simulink model "thermal_closed_loop_model"  (R2023a)
settings: Solver=ode23t  StartTime=0.0  StopTime=600  RelTol=1e-3
PostLoadFcn:
  | run('thermal_model_parameters.m')
  | run('thermal_harness_parameters.m')
  | run('thermal_variants_config.m')
values from neighbouring files (symbols this model uses):
  air_cp = 1004    [cathode_subsystem_parameters.m]    (also in thermal_subsystem_parameters.m)
  air_HC_min = 10    [cathode_subsystem_parameters.m]    (also in thermal_subsystem_parameters.m)
  air_HC_nom = 100    [cathode_subsystem_parameters.m]    (also in thermal_subsystem_parameters.m)
  air_rho = 1.2    [cathode_subsystem_parameters.m]    (also in thermal_subsystem_parameters.m)
  air_vel_nom = 1    [cathode_subsystem_parameters.m]    (also in thermal_subsystem_parameters.m)
  coolant_initial_pressure = 0.111325    [cathode_subsystem_parameters.m]    (also in thermal_subsystem_parameters.m)
  coolant_initial_temperature = 293.15    [cathode_subsystem_parameters.m]    (also in thermal_subsystem_parameters.m)
  coolant_tube_D = 0.05    [cathode_subsystem_parameters.m]    (also in thermal_subsystem_parameters.m)
  Hydrowell_VTS =     [Hydrowell_values_VLV.mat]
  radiator_area_air = 0.10260000000000001    (= 0.1026)    [cathode_subsystem_parameters.m]    (also in thermal_subsystem_parameters.m)
  radiator_area_fins = 2.5436250000000005    (= 2.543625)    [cathode_subsystem_parameters.m]    (also in thermal_subsystem_parameters.m)
  radiator_area_primary = 0.44452500000000011    (= 0.444525)    [cathode_subsystem_parameters.m]    (also in thermal_subsystem_parameters.m = 2 * radiator_tube_length * radiator_width * (radiator_fin_ro)
  radiator_n_tubes = 20    [cathode_subsystem_parameters.m]    (also in thermal_subsystem_parameters.m)
  radiator_tube_height = 0.0015    [cathode_subsystem_parameters.m]    (also in thermal_subsystem_parameters.m)
  radiator_tube_length = 0.45    [cathode_subsystem_parameters.m]    (also in thermal_subsystem_parameters.m)
  radiator_width = 0.025    [cathode_subsystem_parameters.m]    (also in thermal_subsystem_parameters.m)
  tcp_time_constant = 2    [cathode_subsystem_parameters.m]    (also in thermal_subsystem_parameters.m)
undefined symbols (not defined in the file or in its folder): sigbuilder_block, stack
libraries: fl_lib x153, nesl_utility x122, SimscapeFluids_lib x16, slpidlib x5, simulink x1
(part 7 of 8)

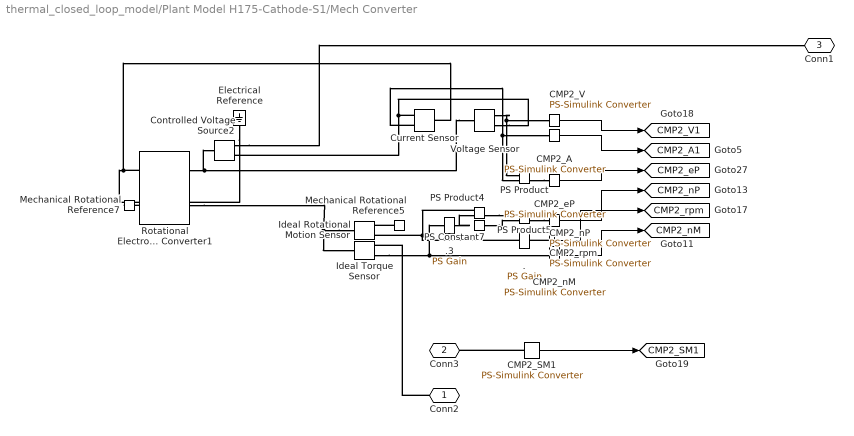
== system thermal_closed_loop_model/Plant Model H175-Cathode-S1/Mech Converter ==
  . : fl_lib/Physical Signals/Functions/PS Gain  gain=1/(0.1047198*1000)
  .3 : fl_lib/Physical Signals/Functions/PS Gain  gain=1/(0.1047198*60)
  CMP2_A : nesl_utility/PS-Simulink Converter  PhysicalDomain=network_engine_domain  SubClassName=ps_output  LeftPortType=input  RightPortType=output  PseudoPeriodic=off  Frequencies=[]  VectorFormat=inherit  Unit=inherit  AffineConversion=off
  CMP2_SM1 : nesl_utility/PS-Simulink Converter  PhysicalDomain=network_engine_domain  SubClassName=ps_output  LeftPortType=input  RightPortType=output  PseudoPeriodic=off  Frequencies=[]  VectorFormat=inherit  Unit=inherit  AffineConversion=off
  CMP2_V : nesl_utility/PS-Simulink Converter  PhysicalDomain=network_engine_domain  SubClassName=ps_output  LeftPortType=input  RightPortType=output  PseudoPeriodic=off  Frequencies=[]  VectorFormat=inherit  Unit=inherit  AffineConversion=off
  CMP2_eP : nesl_utility/PS-Simulink Converter  PhysicalDomain=network_engine_domain  SubClassName=ps_output  LeftPortType=input  RightPortType=output  PseudoPeriodic=off  Frequencies=[]  VectorFormat=inherit  Unit=inherit  AffineConversion=off
  CMP2_nM : nesl_utility/PS-Simulink Converter  PhysicalDomain=network_engine_domain  SubClassName=ps_output  LeftPortType=input  RightPortType=output  PseudoPeriodic=off  Frequencies=[]  VectorFormat=1-D array  Unit=inherit  AffineConversion=off
  CMP2_nP : nesl_utility/PS-Simulink Converter  PhysicalDomain=network_engine_domain  SubClassName=ps_output  LeftPortType=input  RightPortType=output  PseudoPeriodic=off  Frequencies=[]  VectorFormat=inherit  Unit=inherit  AffineConversion=off
  CMP2_rpm : nesl_utility/PS-Simulink Converter  PhysicalDomain=network_engine_domain  SubClassName=ps_output  LeftPortType=input  RightPortType=output  PseudoPeriodic=off  Frequencies=[]  VectorFormat=inherit  Unit=inherit  AffineConversion=off
  Controlled Voltage Source2 : fl_lib/Electrical/Electrical Sources/Controlled Voltage Source
  Current Sensor : fl_lib/Electrical/Electrical Sensors/Current Sensor
  Electrical Reference : fl_lib/Electrical/Electrical Elements/Electrical Reference
  Ideal Rotational Motion Sensor : fl_lib/Mechanical/Mechanical Sensors/Ideal Rotational Motion Sensor  reference=foundation.enum.MeasurementReference.difference  acceleration_port=false  velocity_port=true  position_port=false  wrap_angle=false  offset=0 rad
      settings: InternalSimscapePortConfiguration="{\"Bottom\":[],\"Left\":[{\"id\":\"R\",\"label\":\"R\",\"type\":\"foundation.mechanical.rotational.rotational\"}],\"Right\":[{\"id\":\"C\",\"label\":\"C\",\"type\":\"foundation.mechanical.rotational.rotational\"},{\"id\":\"W\",\"label\":\"W\",\"type\":\"output\"}],\"Top\":[]}"
  Ideal Torque Sensor : fl_lib/Mechanical/Mechanical Sensors/Ideal Torque Sensor
  Mechanical Rotational Reference5 : fl_lib/Mechanical/Rotational Elements/Mechanical Rotational Reference
  Mechanical Rotational Reference7 : fl_lib/Mechanical/Rotational Elements/Mechanical Rotational Reference
  PS Constant7 : fl_lib/Physical Signals/Sources/PS Constant  constant=2*pi
  PS Product : fl_lib/Physical Signals/Functions/PS Product
  PS Product4 : fl_lib/Physical Signals/Functions/PS Product
  PS Product5 : fl_lib/Physical Signals/Functions/PS Product
  Rotational Electromechanical Converter1 : fl_lib/Electrical/Electrical Elements/Rotational Electromechanical Converter  K=0.00409090909090909090909090909091 V/rpm  i_specify=off  i_priority=None  i=0 A  i_nominal_specify=off  i_nominal_unit=A  i_nominal_value=1  v_specify=off  v_priority=None  v=50 V  v_nominal_specify=off  v_nominal_unit=V  v_nominal_value=1  t_specify=off  t_priority=None  t=0 N*m  t_nominal_specify=off  t_nominal_unit=N*m  t_nominal_value=1  w_specify=off  w_priority=None  w=0 rad/s  w_nominal_specify=off  w_nominal_unit=rad/s  w_nominal_value=1
  Voltage Sensor : fl_lib/Electrical/Electrical Sensors/Voltage Sensor
  Conn2 : PMIOPort  Side=Left
  Conn3 : PMIOPort  Port=2  Side=Right
  Conn1 : PMIOPort  Port=3  Side=Right
  tag scope: CMP2_A1=global, CMP2_SM1=global, CMP2_V1=global, CMP2_eP=global, CMP2_nM=global, CMP2_nP=global, CMP2_rpm=global
  wires:
  CMP2_eP/1 -> [CMP2_eP]
  CMP2_V/1 -> [CMP2_V1]
  CMP2_A/1 -> [CMP2_A1]
  CMP2_nM/1 -> [CMP2_nM]
  CMP2_rpm/1 -> [CMP2_rpm]
  CMP2_nP/1 -> [CMP2_nP]
  CMP2_SM1/1 -> [CMP2_SM1]
  connections:
  CMP2_rpm/LConn1 -- ./RConn1
  PS Constant7/RConn1 -- PS Product5/LConn2
  Rotational Electromechanical Converter1/RConn2 -- Mechanical Rotational Reference7/LConn1
  Voltage Sensor/LConn1 -- Controlled Voltage Source2/LConn1 -- Rotational Electromechanical Converter1/LConn1
  Electrical Reference/LConn1 -- Current Sensor/LConn1 -- Rotational Electromechanical Converter1/RConn1
  Current Sensor/RConn1 -- PS Product/LConn1 -- CMP2_A/LConn1
  Controlled Voltage Source2/RConn1 -- Conn1/RConn1
  Ideal Rotational Motion Sensor/LConn1 -- Rotational Electromechanical Converter1/LConn2 -- Ideal Torque Sensor/LConn1
  Current Sensor/RConn2 -- Voltage Sensor/RConn2 -- Controlled Voltage Source2/RConn2
  PS Product/RConn1 -- CMP2_eP/LConn1
  .3/RConn1 -- PS Product4/LConn2
  PS Product4/RConn1 -- PS Product5/LConn1
  Ideal Torque Sensor/RConn2 -- CMP2_nM/LConn1 -- .3/LConn1
  PS Product5/RConn1 -- CMP2_nP/LConn1
  Voltage Sensor/RConn1 -- PS Product/LConn2 -- CMP2_V/LConn1
  ./LConn1 -- PS Product4/LConn1 -- Ideal Rotational Motion Sensor/RConn2
  Mechanical Rotational Reference5/LConn1 -- Ideal Rotational Motion Sensor/RConn1
  Conn2/RConn1 -- Ideal Torque Sensor/RConn1
  CMP2_SM1/LConn1 -- Conn3/RConn1

== system thermal_closed_loop_model/Plant Model H175-Cathode-S1/S1 ==
  Absolute Reference (G) : fl_lib/Gas/Elements/Absolute Reference (G)
      settings: InternalSimscapePortConfiguration="{\"Bottom\":[],\"Left\":[{\"id\":\"A\",\"label\":\"\",\"type\":\"foundation.gas.gas\"}],\"Right\":[],\"Top\":[]}"
  Bus Creator : BusCreator  Inputs=3
  Mass & Energy Flow Rate Sensor (G) : fl_lib/Gas/Sensors/Flow Rate Sensor (G)  mass_flow_measure=true  volumetric_flow_measure=false  volumetric_flow_conditions=foundation.enum.volumetric_flow_conditions.actual  p_std=0.101325 MPa  T_std=20 degC  energy_flow_measure=true
      settings: InternalSimscapePortConfiguration="{\"Bottom\":[{\"id\":\"PHI\",\"label\":\"φ\",\"type\":\"output\"}],\"Left\":[{\"id\":\"A\",\"label\":\"A\",\"type\":\"foundation.gas.gas\"}],\"Right\":[{\"id\":\"B\",\"label\":\"B\",\"type\":\"foundation.gas.gas\"},{\"id\":\"M\",\"label\":\"M\",\"type\":\"output\"}],\"Top\":[]}"
  Pressure & Temperature Sensor (G)4 : fl_lib/Gas/Sensors/Pressure & Temperature Sensor (G)  reference=foundation.enum.MeasurementReference.difference  pressure=true  pressure_spec=foundation.enum.PressureMeasementSpec.Absolute  temperature=true
      settings: InternalSimscapePortConfiguration="{\"Bottom\":[{\"id\":\"T\",\"label\":\"T\",\"type\":\"output\"}],\"Left\":[{\"id\":\"A\",\"label\":\"A\",\"type\":\"foundation.gas.gas\"}],\"Right\":[{\"id\":\"B\",\"label\":\"B\",\"type\":\"foundation.gas.gas\"},{\"id\":\"P\",\"label\":\"P\",\"type\":\"output\"}],\"Top\":[]}"
  aPres_S1 : nesl_utility/PS-Simulink Converter  PhysicalDomain=network_engine_domain  SubClassName=ps_output  LeftPortType=input  RightPortType=output  PseudoPeriodic=off  Frequencies=[]  VectorFormat=inherit  Unit=inherit  AffineConversion=off
  aTemp_S1 : nesl_utility/PS-Simulink Converter  PhysicalDomain=network_engine_domain  SubClassName=ps_output  LeftPortType=input  RightPortType=output  PseudoPeriodic=off  Frequencies=[]  VectorFormat=inherit  Unit=degC  AffineConversion=off
  aTemp_S2 : nesl_utility/PS-Simulink Converter  PhysicalDomain=network_engine_domain  SubClassName=ps_output  LeftPortType=input  RightPortType=output  PseudoPeriodic=off  Frequencies=[]  VectorFormat=inherit  Unit=inherit  AffineConversion=off
  Conn1 : PMIOPort  Side=Left
  Conn2 : PMIOPort  Port=2  Side=Right
  tag scope: S1=global
  wires:
  aTemp_S1/1 -> Bus Creator/2  "aTemp_S1"
  aPres_S1/1 -> Bus Creator/1  "aPres_S1"
  aTemp_S2/1 -> Bus Creator/3  "mFlow_S1"
  Bus Creator/1 -> [S1]
  connections:
  Absolute Reference (G)/LConn1 -- Pressure & Temperature Sensor (G)4/RConn1
  aPres_S1/LConn1 -- Pressure & Temperature Sensor (G)4/RConn2
  aTemp_S1/LConn1 -- Pressure & Temperature Sensor (G)4/RConn3
  Pressure & Temperature Sensor (G)4/LConn1 -- Mass & Energy Flow Rate Sensor (G)/LConn1 -- Conn1/RConn1
  Mass & Energy Flow Rate Sensor (G)/RConn2 -- aTemp_S2/LConn1
  Mass & Energy Flow Rate Sensor (G)/RConn1 -- Conn2/RConn1

== system thermal_closed_loop_model/Plant Model H175-Cathode-S1/S2 ==
  Absolute Reference (G) : fl_lib/Gas/Elements/Absolute Reference (G)
      settings: InternalSimscapePortConfiguration="{\"Bottom\":[],\"Left\":[{\"id\":\"A\",\"label\":\"\",\"type\":\"foundation.gas.gas\"}],\"Right\":[],\"Top\":[]}"
  Bus Creator : BusCreator  Inputs=3
  Mass & Energy Flow Rate Sensor (G) : fl_lib/Gas/Sensors/Flow Rate Sensor (G)  mass_flow_measure=true  volumetric_flow_measure=false  volumetric_flow_conditions=foundation.enum.volumetric_flow_conditions.actual  p_std=0.101325 MPa  T_std=20 degC  energy_flow_measure=true
      settings: InternalSimscapePortConfiguration="{\"Bottom\":[{\"id\":\"PHI\",\"label\":\"φ\",\"type\":\"output\"}],\"Left\":[{\"id\":\"A\",\"label\":\"A\",\"type\":\"foundation.gas.gas\"}],\"Right\":[{\"id\":\"B\",\"label\":\"B\",\"type\":\"foundation.gas.gas\"},{\"id\":\"M\",\"label\":\"M\",\"type\":\"output\"}],\"Top\":[]}"
  Pressure & Temperature Sensor (G)4 : fl_lib/Gas/Sensors/Pressure & Temperature Sensor (G)  reference=foundation.enum.MeasurementReference.difference  pressure=true  pressure_spec=foundation.enum.PressureMeasementSpec.Absolute  temperature=true
      settings: InternalSimscapePortConfiguration="{\"Bottom\":[{\"id\":\"T\",\"label\":\"T\",\"type\":\"output\"}],\"Left\":[{\"id\":\"A\",\"label\":\"A\",\"type\":\"foundation.gas.gas\"}],\"Right\":[{\"id\":\"B\",\"label\":\"B\",\"type\":\"foundation.gas.gas\"},{\"id\":\"P\",\"label\":\"P\",\"type\":\"output\"}],\"Top\":[]}"
  To Workspace : ToWorkspace  VariableName=EAC_aPres_S2  SaveFormat=Timeseries  SampleTime=-1
  aPres_S1 : nesl_utility/PS-Simulink Converter  PhysicalDomain=network_engine_domain  SubClassName=ps_output  LeftPortType=input  RightPortType=output  PseudoPeriodic=off  Frequencies=[]  VectorFormat=inherit  Unit=inherit  AffineConversion=off
  aTemp_S1 : nesl_utility/PS-Simulink Converter  PhysicalDomain=network_engine_domain  SubClassName=ps_output  LeftPortType=input  RightPortType=output  PseudoPeriodic=off  Frequencies=[]  VectorFormat=inherit  Unit=degC  AffineConversion=off
  mFlow_S2 : nesl_utility/PS-Simulink Converter  PhysicalDomain=network_engine_domain  SubClassName=ps_output  LeftPortType=input  RightPortType=output  PseudoPeriodic=off  Frequencies=[]  VectorFormat=inherit  Unit=kg/s  AffineConversion=off
  Conn1 : PMIOPort  Side=Left
  Conn2 : PMIOPort  Port=2  Side=Right
  tag scope: S2=global
  wires:
  aPres_S1/1 -> To Workspace/1, Bus Creator/1  "aPres_S2"
  aTemp_S1/1 -> Bus Creator/2  "aTemp_S2"
  mFlow_S2/1 -> Bus Creator/3  "mFlow_S2"
  Bus Creator/1 -> [S2]
  connections:
  Pressure & Temperature Sensor (G)4/LConn1 -- Mass & Energy Flow Rate Sensor (G)/LConn1 -- Conn1/RConn1
  Absolute Reference (G)/LConn1 -- Pressure & Temperature Sensor (G)4/RConn1
  aPres_S1/LConn1 -- Pressure & Temperature Sensor (G)4/RConn2
  aTemp_S1/LConn1 -- Pressure & Temperature Sensor (G)4/RConn3
  Mass & Energy Flow Rate Sensor (G)/RConn1 -- Conn2/RConn1
  Mass & Energy Flow Rate Sensor (G)/RConn2 -- mFlow_S2/LConn1

== system thermal_closed_loop_model/Plant Model H175-Cathode-S1/S3 ==
  Absolute Reference (MA) : fl_lib/Moist Air/Elements/Absolute Reference (MA)
  Bus Creator : BusCreator  Inputs=9
  Humidity & Trace Gas Sensor (MA)1 : fl_lib/Moist Air/Sensors/Humidity & Trace Gas Sensor (MA)  moisture_on=true  moisture_spec=foundation.enum.moisture_spec.relative_humidity  trace_gas_on=true  trace_gas_spec=foundation.enum.trace_gas_spec.mass_fraction
      settings: InternalSimscapePortConfiguration="{\"Bottom\":[],\"Left\":[{\"id\":\"A\",\"label\":\"A\",\"type\":\"foundation.moist_air.moist_air\"}],\"Right\":[{\"id\":\"W\",\"label\":\"W\",\"type\":\"output\"},{\"id\":\"G\",\"label\":\"G\",\"type\":\"output\"}],\"Top\":[]}"
  Mass & Energy Flow Rate Sensor (MA) : fl_lib/Moist Air/Sensors/Flow Rate Sensor (MA)  mass_flow_measure=true  volumetric_flow_measure=false  volumetric_flow_conditions=foundation.enum.volumetric_flow_conditions.actual  p_std=0.101325 MPa  T_std=20 degC  RH_std=0.65  energy_flow_measure=true  vapor_flow_measure=true  gas_flow_measure=true
      settings: InternalSimscapePortConfiguration="{\"Bottom\":[{\"id\":\"PHI\",\"label\":\"φ\",\"type\":\"output\"}],\"Left\":[{\"id\":\"A\",\"label\":\"A\",\"type\":\"foundation.moist_air.moist_air\"},{\"id\":\"Mw\",\"label\":\"Mw\",\"type\":\"output\"},{\"id\":\"Mg\",\"label\":\"Mg\",\"type\":\"output\"}],\"Right\":[{\"id\":\"B\",\"label\":\"B\",\"type\":\"foundation.moist_air.moist_air\"},{\"id\":\"M\",\"label\":\"M\",\"type\":\"output\"}],\"Top\":[]}"
  MixDensity : nesl_utility/PS-Simulink Converter  PhysicalDomain=network_engine_domain  SubClassName=ps_output  LeftPortType=input  RightPortType=output  PseudoPeriodic=off  Frequencies=[]  VectorFormat=inherit  Unit=inherit  AffineConversion=off
  MixSEnthaply : nesl_utility/PS-Simulink Converter  PhysicalDomain=network_engine_domain  SubClassName=ps_output  LeftPortType=input  RightPortType=output  PseudoPeriodic=off  Frequencies=[]  VectorFormat=inherit  Unit=inherit  AffineConversion=off
  Pressure & Temperature Sensor (MA) : fl_lib/Moist Air/Sensors/Pressure & Temperature Sensor (MA)  reference=foundation.enum.MeasurementReference.difference  pressure=true  pressure_spec=foundation.enum.PressureMeasementSpec.Absolute  temperature=true
      settings: InternalSimscapePortConfiguration="{\"Bottom\":[{\"id\":\"T\",\"label\":\"T\",\"type\":\"output\"}],\"Left\":[{\"id\":\"A\",\"label\":\"A\",\"type\":\"foundation.moist_air.moist_air\"}],\"Right\":[{\"id\":\"B\",\"label\":\"B\",\"type\":\"foundation.moist_air.moist_air\"},{\"id\":\"P\",\"label\":\"P\",\"type\":\"output\"}],\"Top\":[]}"
  SEntropy : nesl_utility/PS-Simulink Converter  PhysicalDomain=network_engine_domain  SubClassName=ps_output  LeftPortType=input  RightPortType=output  PseudoPeriodic=off  Frequencies=[]  VectorFormat=inherit  Unit=inherit  AffineConversion=off
  SHeat : nesl_utility/PS-Simulink Converter  PhysicalDomain=network_engine_domain  SubClassName=ps_output  LeftPortType=input  RightPortType=output  PseudoPeriodic=off  Frequencies=[]  VectorFormat=inherit  Unit=inherit  AffineConversion=off
  Thermodynamic Properties Sensor (MA) : fl_lib/Moist Air/Sensors/Thermodynamic Properties Sensor (MA)  measurement_mass_spec=foundation.enum.measurement_mass_spec.mixture  enthalpy=true  density=true  specific_heat=true  entropy=true
      settings: InternalSimscapePortConfiguration="{\"Bottom\":[{\"id\":\"CP\",\"label\":\"cp\",\"type\":\"output\"},{\"id\":\"S\",\"label\":\"s\",\"type\":\"output\"}],\"Left\":[{\"id\":\"A\",\"label\":\"A\",\"type\":\"foundation.moist_air.moist_air\"}],\"Right\":[{\"id\":\"H\",\"label\":\"h\",\"type\":\"output\"},{\"id\":\"RHO\",\"label\":\"ρ\",\"type\":\"output\"}],\"Top\":[]}"
  aPres_S4 : nesl_utility/PS-Simulink Converter  PhysicalDomain=network_engine_domain  SubClassName=ps_output  LeftPortType=input  RightPortType=output  PseudoPeriodic=off  Frequencies=[]  VectorFormat=inherit  Unit=inherit  AffineConversion=off
  aTemp : nesl_utility/PS-Simulink Converter  PhysicalDomain=network_engine_domain  SubClassName=ps_output  LeftPortType=input  RightPortType=output  PseudoPeriodic=off  Frequencies=[]  VectorFormat=inherit  Unit=inherit  AffineConversion=off
  mFlow : nesl_utility/PS-Simulink Converter  PhysicalDomain=network_engine_domain  SubClassName=ps_output  LeftPortType=input  RightPortType=output  PseudoPeriodic=off  Frequencies=[]  VectorFormat=inherit  Unit=inherit  AffineConversion=off
  mFraction : nesl_utility/PS-Simulink Converter  PhysicalDomain=network_engine_domain  SubClassName=ps_output  LeftPortType=input  RightPortType=output  PseudoPeriodic=off  Frequencies=[]  VectorFormat=inherit  Unit=inherit  AffineConversion=off
  relHum : nesl_utility/PS-Simulink Converter  PhysicalDomain=network_engine_domain  SubClassName=ps_output  LeftPortType=input  RightPortType=output  PseudoPeriodic=off  Frequencies=[]  VectorFormat=inherit  Unit=inherit  AffineConversion=off
  Conn2 : PMIOPort  Side=Left
  Conn1 : PMIOPort  Port=2  Side=Right
  tag scope: S3=global
  wires:
  aTemp/1 -> Bus Creator/2  "aTemp_S3"
  aPres_S4/1 -> Bus Creator/1  "aPres_S3"
  SEntropy/1 -> Bus Creator/9  "SEntropy_S3"
  MixSEnthaply/1 -> Bus Creator/6  "MixSEnthalpy_S3"
  MixDensity/1 -> Bus Creator/7  "MixDensity_S3"
  mFraction/1 -> Bus Creator/5  "mFraction_S3"
  mFlow/1 -> Bus Creator/3  "mFlow_S3"
  relHum/1 -> Bus Creator/4  "relHum_S3"
  SHeat/1 -> Bus Creator/8  "SHeat_S3"
  Bus Creator/1 -> [S3]
  connections:
  Mass & Energy Flow Rate Sensor (MA)/LConn1 -- Conn1/RConn1
  Humidity & Trace Gas Sensor (MA)1/RConn1 -- relHum/LConn1
  MixSEnthaply/LConn1 -- Thermodynamic Properties Sensor (MA)/RConn1
  MixDensity/LConn1 -- Thermodynamic Properties Sensor (MA)/RConn2
  SHeat/LConn1 -- Thermodynamic Properties Sensor (MA)/RConn4
  aTemp/LConn1 -- Pressure & Temperature Sensor (MA)/RConn3
  SEntropy/LConn1 -- Thermodynamic Properties Sensor (MA)/RConn3
  Conn2/RConn1 -- Mass & Energy Flow Rate Sensor (MA)/RConn1 -- Thermodynamic Properties Sensor (MA)/LConn1 -- Pressure & Temperature Sensor (MA)/LConn1 -- Humidity & Trace Gas Sensor (MA)1/LConn1
  mFlow/LConn1 -- Mass & Energy Flow Rate Sensor (MA)/RConn2
  Pressure & Temperature Sensor (MA)/RConn2 -- aPres_S4/LConn1
  Humidity & Trace Gas Sensor (MA)1/RConn2 -- mFraction/LConn1
  Absolute Reference (MA)/LConn1 -- Pressure & Temperature Sensor (MA)/RConn1

== system thermal_closed_loop_model/Plant Model H175-Cathode-S1/S4 ==
  Absolute Reference (MA) : fl_lib/Moist Air/Elements/Absolute Reference (MA)
  Bus Creator : BusCreator  Inputs=9
  Humidity & Trace Gas Sensor (MA)1 : fl_lib/Moist Air/Sensors/Humidity & Trace Gas Sensor (MA)  moisture_on=true  moisture_spec=foundation.enum.moisture_spec.relative_humidity  trace_gas_on=true  trace_gas_spec=foundation.enum.trace_gas_spec.mass_fraction
      settings: InternalSimscapePortConfiguration="{\"Bottom\":[],\"Left\":[{\"id\":\"A\",\"label\":\"A\",\"type\":\"foundation.moist_air.moist_air\"}],\"Right\":[{\"id\":\"W\",\"label\":\"W\",\"type\":\"output\"},{\"id\":\"G\",\"label\":\"G\",\"type\":\"output\"}],\"Top\":[]}"
  Mass & Energy Flow Rate Sensor (MA) : fl_lib/Moist Air/Sensors/Flow Rate Sensor (MA)  mass_flow_measure=true  volumetric_flow_measure=false  volumetric_flow_conditions=foundation.enum.volumetric_flow_conditions.actual  p_std=0.101325 MPa  T_std=20 degC  RH_std=0.65  energy_flow_measure=true  vapor_flow_measure=true  gas_flow_measure=true
      settings: InternalSimscapePortConfiguration="{\"Bottom\":[{\"id\":\"PHI\",\"label\":\"φ\",\"type\":\"output\"}],\"Left\":[{\"id\":\"A\",\"label\":\"A\",\"type\":\"foundation.moist_air.moist_air\"},{\"id\":\"Mw\",\"label\":\"Mw\",\"type\":\"output\"},{\"id\":\"Mg\",\"label\":\"Mg\",\"type\":\"output\"}],\"Right\":[{\"id\":\"B\",\"label\":\"B\",\"type\":\"foundation.moist_air.moist_air\"},{\"id\":\"M\",\"label\":\"M\",\"type\":\"output\"}],\"Top\":[]}"
  MixDensity : nesl_utility/PS-Simulink Converter  PhysicalDomain=network_engine_domain  SubClassName=ps_output  LeftPortType=input  RightPortType=output  PseudoPeriodic=off  Frequencies=[]  VectorFormat=inherit  Unit=inherit  AffineConversion=off
  MixSEnthaply : nesl_utility/PS-Simulink Converter  PhysicalDomain=network_engine_domain  SubClassName=ps_output  LeftPortType=input  RightPortType=output  PseudoPeriodic=off  Frequencies=[]  VectorFormat=inherit  Unit=inherit  AffineConversion=off
  Pressure & Temperature Sensor (MA) : fl_lib/Moist Air/Sensors/Pressure & Temperature Sensor (MA)  reference=foundation.enum.MeasurementReference.difference  pressure=true  pressure_spec=foundation.enum.PressureMeasementSpec.Absolute  temperature=true
      settings: InternalSimscapePortConfiguration="{\"Bottom\":[{\"id\":\"T\",\"label\":\"T\",\"type\":\"output\"}],\"Left\":[{\"id\":\"A\",\"label\":\"A\",\"type\":\"foundation.moist_air.moist_air\"}],\"Right\":[{\"id\":\"B\",\"label\":\"B\",\"type\":\"foundation.moist_air.moist_air\"},{\"id\":\"P\",\"label\":\"P\",\"type\":\"output\"}],\"Top\":[]}"
  SEntropy : nesl_utility/PS-Simulink Converter  PhysicalDomain=network_engine_domain  SubClassName=ps_output  LeftPortType=input  RightPortType=output  PseudoPeriodic=off  Frequencies=[]  VectorFormat=inherit  Unit=inherit  AffineConversion=off
  SHeat : nesl_utility/PS-Simulink Converter  PhysicalDomain=network_engine_domain  SubClassName=ps_output  LeftPortType=input  RightPortType=output  PseudoPeriodic=off  Frequencies=[]  VectorFormat=inherit  Unit=inherit  AffineConversion=off
  Thermodynamic Properties Sensor (MA) : fl_lib/Moist Air/Sensors/Thermodynamic Properties Sensor (MA)  measurement_mass_spec=foundation.enum.measurement_mass_spec.mixture  enthalpy=true  density=true  specific_heat=true  entropy=true
      settings: InternalSimscapePortConfiguration="{\"Bottom\":[{\"id\":\"CP\",\"label\":\"cp\",\"type\":\"output\"},{\"id\":\"S\",\"label\":\"s\",\"type\":\"output\"}],\"Left\":[{\"id\":\"A\",\"label\":\"A\",\"type\":\"foundation.moist_air.moist_air\"}],\"Right\":[{\"id\":\"H\",\"label\":\"h\",\"type\":\"output\"},{\"id\":\"RHO\",\"label\":\"ρ\",\"type\":\"output\"}],\"Top\":[]}"
  aPres_S4 : nesl_utility/PS-Simulink Converter  PhysicalDomain=network_engine_domain  SubClassName=ps_output  LeftPortType=input  RightPortType=output  PseudoPeriodic=off  Frequencies=[]  VectorFormat=inherit  Unit=inherit  AffineConversion=off
  aTemp : nesl_utility/PS-Simulink Converter  PhysicalDomain=network_engine_domain  SubClassName=ps_output  LeftPortType=input  RightPortType=output  PseudoPeriodic=off  Frequencies=[]  VectorFormat=inherit  Unit=inherit  AffineConversion=off
  mFlow : nesl_utility/PS-Simulink Converter  PhysicalDomain=network_engine_domain  SubClassName=ps_output  LeftPortType=input  RightPortType=output  PseudoPeriodic=off  Frequencies=[]  VectorFormat=inherit  Unit=inherit  AffineConversion=off
  mFraction : nesl_utility/PS-Simulink Converter  PhysicalDomain=network_engine_domain  SubClassName=ps_output  LeftPortType=input  RightPortType=output  PseudoPeriodic=off  Frequencies=[]  VectorFormat=inherit  Unit=inherit  AffineConversion=off
  relHum : nesl_utility/PS-Simulink Converter  PhysicalDomain=network_engine_domain  SubClassName=ps_output  LeftPortType=input  RightPortType=output  PseudoPeriodic=off  Frequencies=[]  VectorFormat=inherit  Unit=inherit  AffineConversion=off
  Conn1 : PMIOPort  Side=Left
  Conn2 : PMIOPort  Port=2  Side=Right
  tag scope: S4=global
  wires:
  SHeat/1 -> Bus Creator/8  "SHeat_S4"
  relHum/1 -> Bus Creator/4  "relHum_S4"
  mFlow/1 -> Bus Creator/3  "mFlow_S4"
  mFraction/1 -> Bus Creator/5  "mFraction_S4"
  MixDensity/1 -> Bus Creator/7  "MixDensity_S4"
  MixSEnthaply/1 -> Bus Creator/6  "MixSEnthalpy_S4"
  SEntropy/1 -> Bus Creator/9  "SEntropy_S4"
  aPres_S4/1 -> Bus Creator/1  "aPres_S4"
  aTemp/1 -> Bus Creator/2  "aTemp_S4"
  Bus Creator/1 -> [S4]
  connections:
  Humidity & Trace Gas Sensor (MA)1/RConn2 -- mFraction/LConn1
  Pressure & Temperature Sensor (MA)/RConn2 -- aPres_S4/LConn1
  Mass & Energy Flow Rate Sensor (MA)/RConn2 -- mFlow/LConn1
  Pressure & Temperature Sensor (MA)/LConn1 -- Thermodynamic Properties Sensor (MA)/LConn1 -- Mass & Energy Flow Rate Sensor (MA)/RConn1 -- Conn2/RConn1 -- Humidity & Trace Gas Sensor (MA)1/LConn1
  SEntropy/LConn1 -- Thermodynamic Properties Sensor (MA)/RConn3
  aTemp/LConn1 -- Pressure & Temperature Sensor (MA)/RConn3
  SHeat/LConn1 -- Thermodynamic Properties Sensor (MA)/RConn4
  MixDensity/LConn1 -- Thermodynamic Properties Sensor (MA)/RConn2
  MixSEnthaply/LConn1 -- Thermodynamic Properties Sensor (MA)/RConn1
  Humidity & Trace Gas Sensor (MA)1/RConn1 -- relHum/LConn1
  Conn1/RConn1 -- Mass & Energy Flow Rate Sensor (MA)/LConn1
  Pressure & Temperature Sensor (MA)/RConn1 -- Absolute Reference (MA)/LConn1

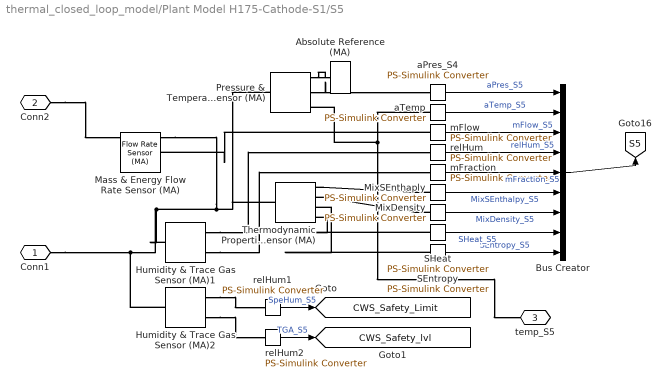
== system thermal_closed_loop_model/Plant Model H175-Cathode-S1/S5 ==
  Absolute Reference (MA) : fl_lib/Moist Air/Elements/Absolute Reference (MA)
  Bus Creator : BusCreator  Inputs=9
  Humidity & Trace Gas Sensor (MA)1 : fl_lib/Moist Air/Sensors/Humidity & Trace Gas Sensor (MA)  moisture_on=true  moisture_spec=foundation.enum.moistureSpec.RelativeHumidity  trace_gas_on=true  trace_gas_spec=foundation.enum.trace_gas_spec.mass_fraction
      settings: InternalSimscapePortConfiguration="{\"Bottom\":[],\"Left\":[{\"id\":\"A\",\"label\":\"A\",\"type\":\"foundation.moist_air.moist_air\"}],\"Right\":[{\"id\":\"W\",\"label\":\"W\",\"type\":\"output\"},{\"id\":\"G\",\"label\":\"G\",\"type\":\"output\"}],\"Top\":[]}"
  Humidity & Trace Gas Sensor (MA)2 : fl_lib/Moist Air/Sensors/Humidity & Trace Gas Sensor (MA)  moisture_on=true  moisture_spec=foundation.enum.moistureSpec.SpecificHumidity  trace_gas_on=true  trace_gas_spec=foundation.enum.trace_gas_spec.mass_fraction
      settings: InternalSimscapePortConfiguration="{\"Bottom\":[],\"Left\":[{\"id\":\"A\",\"label\":\"A\",\"type\":\"foundation.moist_air.moist_air\"}],\"Right\":[{\"id\":\"W\",\"label\":\"W\",\"type\":\"output\"},{\"id\":\"G\",\"label\":\"G\",\"type\":\"output\"}],\"Top\":[]}"
  Mass & Energy Flow Rate Sensor (MA) : fl_lib/Moist Air/Sensors/Flow Rate Sensor (MA)  mass_flow_measure=true  volumetric_flow_measure=false  volumetric_flow_conditions=foundation.enum.volumetric_flow_conditions.actual  p_std=0.101325 MPa  T_std=20 degC  RH_std=0.65  energy_flow_measure=true  vapor_flow_measure=true  gas_flow_measure=true
      settings: InternalSimscapePortConfiguration="{\"Bottom\":[{\"id\":\"PHI\",\"label\":\"φ\",\"type\":\"output\"}],\"Left\":[{\"id\":\"A\",\"label\":\"A\",\"type\":\"foundation.moist_air.moist_air\"},{\"id\":\"Mw\",\"label\":\"Mw\",\"type\":\"output\"},{\"id\":\"Mg\",\"label\":\"Mg\",\"type\":\"output\"}],\"Right\":[{\"id\":\"B\",\"label\":\"B\",\"type\":\"foundation.moist_air.moist_air\"},{\"id\":\"M\",\"label\":\"M\",\"type\":\"output\"}],\"Top\":[]}"
  MixDensity : nesl_utility/PS-Simulink Converter  PhysicalDomain=network_engine_domain  SubClassName=ps_output  LeftPortType=input  RightPortType=output  PseudoPeriodic=off  Frequencies=[]  VectorFormat=inherit  Unit=inherit  AffineConversion=off
  MixSEnthaply : nesl_utility/PS-Simulink Converter  PhysicalDomain=network_engine_domain  SubClassName=ps_output  LeftPortType=input  RightPortType=output  PseudoPeriodic=off  Frequencies=[]  VectorFormat=inherit  Unit=inherit  AffineConversion=off
  Pressure & Temperature Sensor (MA) : fl_lib/Moist Air/Sensors/Pressure & Temperature Sensor (MA)  reference=foundation.enum.MeasurementReference.difference  pressure=true  pressure_spec=foundation.enum.PressureMeasementSpec.Absolute  temperature=true
      settings: InternalSimscapePortConfiguration="{\"Bottom\":[{\"id\":\"T\",\"label\":\"T\",\"type\":\"output\"}],\"Left\":[{\"id\":\"A\",\"label\":\"A\",\"type\":\"foundation.moist_air.moist_air\"}],\"Right\":[{\"id\":\"B\",\"label\":\"B\",\"type\":\"foundation.moist_air.moist_air\"},{\"id\":\"P\",\"label\":\"P\",\"type\":\"output\"}],\"Top\":[]}"
  SEntropy : nesl_utility/PS-Simulink Converter  PhysicalDomain=network_engine_domain  SubClassName=ps_output  LeftPortType=input  RightPortType=output  PseudoPeriodic=off  Frequencies=[]  VectorFormat=inherit  Unit=inherit  AffineConversion=off
  SHeat : nesl_utility/PS-Simulink Converter  PhysicalDomain=network_engine_domain  SubClassName=ps_output  LeftPortType=input  RightPortType=output  PseudoPeriodic=off  Frequencies=[]  VectorFormat=inherit  Unit=inherit  AffineConversion=off
  Thermodynamic Properties Sensor (MA) : fl_lib/Moist Air/Sensors/Thermodynamic Properties Sensor (MA)  measurement_mass_spec=foundation.enum.measurement_mass_spec.mixture  enthalpy=true  density=true  specific_heat=true  entropy=true
      settings: InternalSimscapePortConfiguration="{\"Bottom\":[{\"id\":\"CP\",\"label\":\"cp\",\"type\":\"output\"},{\"id\":\"S\",\"label\":\"s\",\"type\":\"output\"}],\"Left\":[{\"id\":\"A\",\"label\":\"A\",\"type\":\"foundation.moist_air.moist_air\"}],\"Right\":[{\"id\":\"H\",\"label\":\"h\",\"type\":\"output\"},{\"id\":\"RHO\",\"label\":\"ρ\",\"type\":\"output\"}],\"Top\":[]}"
  aPres_S4 : nesl_utility/PS-Simulink Converter  PhysicalDomain=network_engine_domain  SubClassName=ps_output  LeftPortType=input  RightPortType=output  PseudoPeriodic=off  Frequencies=[]  VectorFormat=inherit  Unit=inherit  AffineConversion=off
  aTemp : nesl_utility/PS-Simulink Converter  PhysicalDomain=network_engine_domain  SubClassName=ps_output  LeftPortType=input  RightPortType=output  PseudoPeriodic=off  Frequencies=[]  VectorFormat=inherit  Unit=inherit  AffineConversion=off
  mFlow : nesl_utility/PS-Simulink Converter  PhysicalDomain=network_engine_domain  SubClassName=ps_output  LeftPortType=input  RightPortType=output  PseudoPeriodic=off  Frequencies=[]  VectorFormat=inherit  Unit=inherit  AffineConversion=off
  mFraction : nesl_utility/PS-Simulink Converter  PhysicalDomain=network_engine_domain  SubClassName=ps_output  LeftPortType=input  RightPortType=output  PseudoPeriodic=off  Frequencies=[]  VectorFormat=inherit  Unit=inherit  AffineConversion=off
  relHum : nesl_utility/PS-Simulink Converter  PhysicalDomain=network_engine_domain  SubClassName=ps_output  LeftPortType=input  RightPortType=output  PseudoPeriodic=off  Frequencies=[]  VectorFormat=inherit  Unit=inherit  AffineConversion=off
  relHum1 : nesl_utility/PS-Simulink Converter  PhysicalDomain=network_engine_domain  SubClassName=ps_output  LeftPortType=input  RightPortType=output  PseudoPeriodic=off  Frequencies=[]  VectorFormat=inherit  Unit=inherit  AffineConversion=off
  relHum2 : nesl_utility/PS-Simulink Converter  PhysicalDomain=network_engine_domain  SubClassName=ps_output  LeftPortType=input  RightPortType=output  PseudoPeriodic=off  Frequencies=[]  VectorFormat=inherit  Unit=inherit  AffineConversion=off
  Conn1 : PMIOPort  Side=Left
  Conn2 : PMIOPort  Port=2  Side=Right
  temp_S5 : PMIOPort  Port=3  Side=Left
  tag scope: CWS_Safety_Limit=global, CWS_Safety_lvl=global, S5=global
  wires:
  aTemp/1 -> Bus Creator/2  "aTemp_S5"
  aPres_S4/1 -> Bus Creator/1  "aPres_S5"
  SEntropy/1 -> Bus Creator/9  "SEntropy_S5"
  MixSEnthaply/1 -> Bus Creator/6  "MixSEnthalpy_S5"
  MixDensity/1 -> Bus Creator/7  "MixDensity_S5"
  mFraction/1 -> Bus Creator/5  "mFraction_S5"
  mFlow/1 -> Bus Creator/3  "mFlow_S5"
  relHum/1 -> Bus Creator/4  "relHum_S5"
  SHeat/1 -> Bus Creator/8  "SHeat_S5"
  Bus Creator/1 -> [S5]
  relHum1/1 -> [CWS_Safety_Limit]  "SpeHum_S5"
  relHum2/1 -> [CWS_Safety_lvl]  "TGA_S5"
  connections:
  Conn2/RConn1 -- Mass & Energy Flow Rate Sensor (MA)/LConn1
  Humidity & Trace Gas Sensor (MA)1/RConn1 -- relHum/LConn1
  MixSEnthaply/LConn1 -- Thermodynamic Properties Sensor (MA)/RConn1
  MixDensity/LConn1 -- Thermodynamic Properties Sensor (MA)/RConn2
  SHeat/LConn1 -- Thermodynamic Properties Sensor (MA)/RConn4
  aTemp/LConn1 -- Pressure & Temperature Sensor (MA)/RConn3 -- temp_S5/RConn1
  SEntropy/LConn1 -- Thermodynamic Properties Sensor (MA)/RConn3
  Conn1/RConn1 -- Humidity & Trace Gas Sensor (MA)2/LConn1 -- Mass & Energy Flow Rate Sensor (MA)/RConn1 -- Thermodynamic Properties Sensor (MA)/LConn1 -- Pressure & Temperature Sensor (MA)/LConn1 -- Humidity & Trace Gas Sensor (MA)1/LConn1
  mFlow/LConn1 -- Mass & Energy Flow Rate Sensor (MA)/RConn2
  Pressure & Temperature Sensor (MA)/RConn2 -- aPres_S4/LConn1
  Humidity & Trace Gas Sensor (MA)1/RConn2 -- mFraction/LConn1
  Pressure & Temperature Sensor (MA)/RConn1 -- Absolute Reference (MA)/LConn1
  Humidity & Trace Gas Sensor (MA)2/RConn1 -- relHum1/LConn1
  Humidity & Trace Gas Sensor (MA)2/RConn2 -- relHum2/LConn1

== system thermal_closed_loop_model/Plant Model H175-Cathode-S1/S6 ==
  Absolute Reference (MA) : fl_lib/Moist Air/Elements/Absolute Reference (MA)
  Bus Creator : BusCreator  Inputs=9
  Humidity & Trace Gas Sensor (MA)1 : fl_lib/Moist Air/Sensors/Humidity & Trace Gas Sensor (MA)  moisture_on=true  moisture_spec=foundation.enum.moisture_spec.relative_humidity  trace_gas_on=true  trace_gas_spec=foundation.enum.trace_gas_spec.mass_fraction
      settings: InternalSimscapePortConfiguration="{\"Bottom\":[],\"Left\":[{\"id\":\"A\",\"label\":\"A\",\"type\":\"foundation.moist_air.moist_air\"}],\"Right\":[{\"id\":\"W\",\"label\":\"W\",\"type\":\"output\"},{\"id\":\"G\",\"label\":\"G\",\"type\":\"output\"}],\"Top\":[]}"
  Mass & Energy Flow Rate Sensor (MA) : fl_lib/Moist Air/Sensors/Flow Rate Sensor (MA)  mass_flow_measure=true  volumetric_flow_measure=false  volumetric_flow_conditions=foundation.enum.volumetric_flow_conditions.actual  p_std=0.101325 MPa  T_std=20 degC  RH_std=0.65  energy_flow_measure=true  vapor_flow_measure=true  gas_flow_measure=true
      settings: InternalSimscapePortConfiguration="{\"Bottom\":[{\"id\":\"PHI\",\"label\":\"φ\",\"type\":\"output\"}],\"Left\":[{\"id\":\"A\",\"label\":\"A\",\"type\":\"foundation.moist_air.moist_air\"},{\"id\":\"Mw\",\"label\":\"Mw\",\"type\":\"output\"},{\"id\":\"Mg\",\"label\":\"Mg\",\"type\":\"output\"}],\"Right\":[{\"id\":\"B\",\"label\":\"B\",\"type\":\"foundation.moist_air.moist_air\"},{\"id\":\"M\",\"label\":\"M\",\"type\":\"output\"}],\"Top\":[]}"
  MixDensity : nesl_utility/PS-Simulink Converter  PhysicalDomain=network_engine_domain  SubClassName=ps_output  LeftPortType=input  RightPortType=output  PseudoPeriodic=off  Frequencies=[]  VectorFormat=inherit  Unit=inherit  AffineConversion=off
  MixSEnthaply : nesl_utility/PS-Simulink Converter  PhysicalDomain=network_engine_domain  SubClassName=ps_output  LeftPortType=input  RightPortType=output  PseudoPeriodic=off  Frequencies=[]  VectorFormat=inherit  Unit=inherit  AffineConversion=off
  Pressure & Temperature Sensor (MA) : fl_lib/Moist Air/Sensors/Pressure & Temperature Sensor (MA)  reference=foundation.enum.MeasurementReference.difference  pressure=true  pressure_spec=foundation.enum.PressureMeasementSpec.Absolute  temperature=true
      settings: InternalSimscapePortConfiguration="{\"Bottom\":[{\"id\":\"T\",\"label\":\"T\",\"type\":\"output\"}],\"Left\":[{\"id\":\"A\",\"label\":\"A\",\"type\":\"foundation.moist_air.moist_air\"}],\"Right\":[{\"id\":\"B\",\"label\":\"B\",\"type\":\"foundation.moist_air.moist_air\"},{\"id\":\"P\",\"label\":\"P\",\"type\":\"output\"}],\"Top\":[]}"
  SEntropy : nesl_utility/PS-Simulink Converter  PhysicalDomain=network_engine_domain  SubClassName=ps_output  LeftPortType=input  RightPortType=output  PseudoPeriodic=off  Frequencies=[]  VectorFormat=inherit  Unit=inherit  AffineConversion=off
  SHeat : nesl_utility/PS-Simulink Converter  PhysicalDomain=network_engine_domain  SubClassName=ps_output  LeftPortType=input  RightPortType=output  PseudoPeriodic=off  Frequencies=[]  VectorFormat=inherit  Unit=inherit  AffineConversion=off
  Thermodynamic Properties Sensor (MA) : fl_lib/Moist Air/Sensors/Thermodynamic Properties Sensor (MA)  measurement_mass_spec=foundation.enum.measurement_mass_spec.mixture  enthalpy=true  density=true  specific_heat=true  entropy=true
      settings: InternalSimscapePortConfiguration="{\"Bottom\":[{\"id\":\"CP\",\"label\":\"cp\",\"type\":\"output\"},{\"id\":\"S\",\"label\":\"s\",\"type\":\"output\"}],\"Left\":[{\"id\":\"A\",\"label\":\"A\",\"type\":\"foundation.moist_air.moist_air\"}],\"Right\":[{\"id\":\"H\",\"label\":\"h\",\"type\":\"output\"},{\"id\":\"RHO\",\"label\":\"ρ\",\"type\":\"output\"}],\"Top\":[]}"
  aPres_S4 : nesl_utility/PS-Simulink Converter  PhysicalDomain=network_engine_domain  SubClassName=ps_output  LeftPortType=input  RightPortType=output  PseudoPeriodic=off  Frequencies=[]  VectorFormat=inherit  Unit=inherit  AffineConversion=off
  aTemp : nesl_utility/PS-Simulink Converter  PhysicalDomain=network_engine_domain  SubClassName=ps_output  LeftPortType=input  RightPortType=output  PseudoPeriodic=off  Frequencies=[]  VectorFormat=inherit  Unit=inherit  AffineConversion=off
  mFlow : nesl_utility/PS-Simulink Converter  PhysicalDomain=network_engine_domain  SubClassName=ps_output  LeftPortType=input  RightPortType=output  PseudoPeriodic=off  Frequencies=[]  VectorFormat=inherit  Unit=inherit  AffineConversion=off
  mFraction : nesl_utility/PS-Simulink Converter  PhysicalDomain=network_engine_domain  SubClassName=ps_output  LeftPortType=input  RightPortType=output  PseudoPeriodic=off  Frequencies=[]  VectorFormat=inherit  Unit=inherit  AffineConversion=off
  relHum : nesl_utility/PS-Simulink Converter  PhysicalDomain=network_engine_domain  SubClassName=ps_output  LeftPortType=input  RightPortType=output  PseudoPeriodic=off  Frequencies=[]  VectorFormat=inherit  Unit=inherit  AffineConversion=off
  Conn1 : PMIOPort  Side=Left
  Conn2 : PMIOPort  Port=2  Side=Right
  tag scope: S6=global
  wires:
  SHeat/1 -> Bus Creator/8  "SHeat_S6"
  relHum/1 -> Bus Creator/4  "relHum_S6"
  mFlow/1 -> Bus Creator/3  "mFlow_S6"
  mFraction/1 -> Bus Creator/5  "mFraction_S6"
  MixDensity/1 -> Bus Creator/7  "MixDensity_S6"
  MixSEnthaply/1 -> Bus Creator/6  "MixSEnthalpy_S6"
  SEntropy/1 -> Bus Creator/9  "SEntropy_S6"
  aPres_S4/1 -> Bus Creator/1  "aPres_S6"
  aTemp/1 -> Bus Creator/2  "aTemp_S6"
  Bus Creator/1 -> [S6]
  connections:
  Humidity & Trace Gas Sensor (MA)1/RConn2 -- mFraction/LConn1
  Pressure & Temperature Sensor (MA)/RConn2 -- aPres_S4/LConn1
  mFlow/LConn1 -- Mass & Energy Flow Rate Sensor (MA)/RConn2
  Conn2/RConn1 -- Mass & Energy Flow Rate Sensor (MA)/LConn1
  SEntropy/LConn1 -- Thermodynamic Properties Sensor (MA)/RConn3
  aTemp/LConn1 -- Pressure & Temperature Sensor (MA)/RConn3
  SHeat/LConn1 -- Thermodynamic Properties Sensor (MA)/RConn4
  MixDensity/LConn1 -- Thermodynamic Properties Sensor (MA)/RConn2
  MixSEnthaply/LConn1 -- Thermodynamic Properties Sensor (MA)/RConn1
  Humidity & Trace Gas Sensor (MA)1/RConn1 -- relHum/LConn1
  Mass & Energy Flow Rate Sensor (MA)/RConn1 -- Conn1/RConn1 -- Pressure & Temperature Sensor (MA)/LConn1 -- Thermodynamic Properties Sensor (MA)/LConn1 -- Humidity & Trace Gas Sensor (MA)1/LConn1
  Absolute Reference (MA)/LConn1 -- Pressure & Temperature Sensor (MA)/RConn1

== system thermal_closed_loop_model/Plant Model H175-Cathode-S1/S7 ==
  Absolute Reference (MA) : fl_lib/Moist Air/Elements/Absolute Reference (MA)
  Bus Creator : BusCreator  Inputs=9
  Humidity & Trace Gas Sensor (MA)1 : fl_lib/Moist Air/Sensors/Humidity & Trace Gas Sensor (MA)  moisture_on=true  moisture_spec=foundation.enum.moisture_spec.relative_humidity  trace_gas_on=true  trace_gas_spec=foundation.enum.trace_gas_spec.mass_fraction
      settings: InternalSimscapePortConfiguration="{\"Bottom\":[],\"Left\":[{\"id\":\"A\",\"label\":\"A\",\"type\":\"foundation.moist_air.moist_air\"}],\"Right\":[{\"id\":\"W\",\"label\":\"W\",\"type\":\"output\"},{\"id\":\"G\",\"label\":\"G\",\"type\":\"output\"}],\"Top\":[]}"
  Mass & Energy Flow Rate Sensor (MA) : fl_lib/Moist Air/Sensors/Flow Rate Sensor (MA)  mass_flow_measure=true  volumetric_flow_measure=false  volumetric_flow_conditions=foundation.enum.volumetric_flow_conditions.actual  p_std=0.101325 MPa  T_std=20 degC  RH_std=0.65  energy_flow_measure=true  vapor_flow_measure=true  gas_flow_measure=true
      settings: InternalSimscapePortConfiguration="{\"Bottom\":[{\"id\":\"PHI\",\"label\":\"φ\",\"type\":\"output\"}],\"Left\":[{\"id\":\"A\",\"label\":\"A\",\"type\":\"foundation.moist_air.moist_air\"},{\"id\":\"Mw\",\"label\":\"Mw\",\"type\":\"output\"},{\"id\":\"Mg\",\"label\":\"Mg\",\"type\":\"output\"}],\"Right\":[{\"id\":\"B\",\"label\":\"B\",\"type\":\"foundation.moist_air.moist_air\"},{\"id\":\"M\",\"label\":\"M\",\"type\":\"output\"}],\"Top\":[]}"
  MixDensity : nesl_utility/PS-Simulink Converter  PhysicalDomain=network_engine_domain  SubClassName=ps_output  LeftPortType=input  RightPortType=output  PseudoPeriodic=off  Frequencies=[]  VectorFormat=inherit  Unit=inherit  AffineConversion=off
  MixSEnthaply : nesl_utility/PS-Simulink Converter  PhysicalDomain=network_engine_domain  SubClassName=ps_output  LeftPortType=input  RightPortType=output  PseudoPeriodic=off  Frequencies=[]  VectorFormat=inherit  Unit=inherit  AffineConversion=off
  Pressure & Temperature Sensor (MA) : fl_lib/Moist Air/Sensors/Pressure & Temperature Sensor (MA)  reference=foundation.enum.MeasurementReference.difference  pressure=true  pressure_spec=foundation.enum.PressureMeasementSpec.Absolute  temperature=true
      settings: InternalSimscapePortConfiguration="{\"Bottom\":[{\"id\":\"T\",\"label\":\"T\",\"type\":\"output\"}],\"Left\":[{\"id\":\"A\",\"label\":\"A\",\"type\":\"foundation.moist_air.moist_air\"}],\"Right\":[{\"id\":\"B\",\"label\":\"B\",\"type\":\"foundation.moist_air.moist_air\"},{\"id\":\"P\",\"label\":\"P\",\"type\":\"output\"}],\"Top\":[]}"
  SEntropy : nesl_utility/PS-Simulink Converter  PhysicalDomain=network_engine_domain  SubClassName=ps_output  LeftPortType=input  RightPortType=output  PseudoPeriodic=off  Frequencies=[]  VectorFormat=inherit  Unit=inherit  AffineConversion=off
  SHeat : nesl_utility/PS-Simulink Converter  PhysicalDomain=network_engine_domain  SubClassName=ps_output  LeftPortType=input  RightPortType=output  PseudoPeriodic=off  Frequencies=[]  VectorFormat=inherit  Unit=inherit  AffineConversion=off
  Thermodynamic Properties Sensor (MA) : fl_lib/Moist Air/Sensors/Thermodynamic Properties Sensor (MA)  measurement_mass_spec=foundation.enum.measurement_mass_spec.mixture  enthalpy=true  density=true  specific_heat=true  entropy=true
      settings: InternalSimscapePortConfiguration="{\"Bottom\":[{\"id\":\"CP\",\"label\":\"cp\",\"type\":\"output\"},{\"id\":\"S\",\"label\":\"s\",\"type\":\"output\"}],\"Left\":[{\"id\":\"A\",\"label\":\"A\",\"type\":\"foundation.moist_air.moist_air\"}],\"Right\":[{\"id\":\"H\",\"label\":\"h\",\"type\":\"output\"},{\"id\":\"RHO\",\"label\":\"ρ\",\"type\":\"output\"}],\"Top\":[]}"
  aPres_S4 : nesl_utility/PS-Simulink Converter  PhysicalDomain=network_engine_domain  SubClassName=ps_output  LeftPortType=input  RightPortType=output  PseudoPeriodic=off  Frequencies=[]  VectorFormat=inherit  Unit=inherit  AffineConversion=off
  aTemp : nesl_utility/PS-Simulink Converter  PhysicalDomain=network_engine_domain  SubClassName=ps_output  LeftPortType=input  RightPortType=output  PseudoPeriodic=off  Frequencies=[]  VectorFormat=inherit  Unit=inherit  AffineConversion=off
  mFlow : nesl_utility/PS-Simulink Converter  PhysicalDomain=network_engine_domain  SubClassName=ps_output  LeftPortType=input  RightPortType=output  PseudoPeriodic=off  Frequencies=[]  VectorFormat=inherit  Unit=inherit  AffineConversion=off
  mFraction : nesl_utility/PS-Simulink Converter  PhysicalDomain=network_engine_domain  SubClassName=ps_output  LeftPortType=input  RightPortType=output  PseudoPeriodic=off  Frequencies=[]  VectorFormat=inherit  Unit=inherit  AffineConversion=off
  relHum : nesl_utility/PS-Simulink Converter  PhysicalDomain=network_engine_domain  SubClassName=ps_output  LeftPortType=input  RightPortType=output  PseudoPeriodic=off  Frequencies=[]  VectorFormat=inherit  Unit=inherit  AffineConversion=off
  Conn1 : PMIOPort  Side=Left
  Conn2 : PMIOPort  Port=2  Side=Right
  tag scope: S7=global
  wires:
  Bus Creator/1 -> [S7]
  aTemp/1 -> Bus Creator/2  "aTemp_S7"
  aPres_S4/1 -> Bus Creator/1  "aPres_S7"
  SEntropy/1 -> Bus Creator/9  "SEntropy_S7"
  MixSEnthaply/1 -> Bus Creator/6  "MixSEnthalpy_S7"
  MixDensity/1 -> Bus Creator/7  "MixDensity_S7"
  mFraction/1 -> Bus Creator/5  "mFraction_S7"
  mFlow/1 -> Bus Creator/3  "mFlow_S7"
  relHum/1 -> Bus Creator/4  "relHum_S7"
  SHeat/1 -> Bus Creator/8  "SHeat_S7"
  connections:
  Absolute Reference (MA)/LConn1 -- Pressure & Temperature Sensor (MA)/RConn1
  Humidity & Trace Gas Sensor (MA)1/LConn1 -- Thermodynamic Properties Sensor (MA)/LConn1 -- Pressure & Temperature Sensor (MA)/LConn1 -- Conn1/RConn1 -- Mass & Energy Flow Rate Sensor (MA)/RConn1
  Humidity & Trace Gas Sensor (MA)1/RConn1 -- relHum/LConn1
  MixSEnthaply/LConn1 -- Thermodynamic Properties Sensor (MA)/RConn1
  MixDensity/LConn1 -- Thermodynamic Properties Sensor (MA)/RConn2
  SHeat/LConn1 -- Thermodynamic Properties Sensor (MA)/RConn4
  aTemp/LConn1 -- Pressure & Temperature Sensor (MA)/RConn3
  SEntropy/LConn1 -- Thermodynamic Properties Sensor (MA)/RConn3
  Conn2/RConn1 -- Mass & Energy Flow Rate Sensor (MA)/LConn1
  mFlow/LConn1 -- Mass & Energy Flow Rate Sensor (MA)/RConn2
  Pressure & Temperature Sensor (MA)/RConn2 -- aPres_S4/LConn1
  Humidity & Trace Gas Sensor (MA)1/RConn2 -- mFraction/LConn1

== system thermal_closed_loop_model/Plant Model H175-Cathode-S1/S8 ==
  Absolute Reference (G) : fl_lib/Gas/Elements/Absolute Reference (G)
      settings: InternalSimscapePortConfiguration="{\"Bottom\":[],\"Left\":[{\"id\":\"A\",\"label\":\"\",\"type\":\"foundation.gas.gas\"}],\"Right\":[],\"Top\":[]}"
  Bus Creator : BusCreator  Inputs=2
  Pressure & Temperature Sensor (G)4 : fl_lib/Gas/Sensors/Pressure & Temperature Sensor (G)  reference=foundation.enum.MeasurementReference.difference  pressure=true  pressure_spec=foundation.enum.PressureMeasementSpec.Absolute  temperature=true
      settings: InternalSimscapePortConfiguration="{\"Bottom\":[{\"id\":\"T\",\"label\":\"T\",\"type\":\"output\"}],\"Left\":[{\"id\":\"A\",\"label\":\"A\",\"type\":\"foundation.gas.gas\"}],\"Right\":[{\"id\":\"B\",\"label\":\"B\",\"type\":\"foundation.gas.gas\"},{\"id\":\"P\",\"label\":\"P\",\"type\":\"output\"}],\"Top\":[]}"
  aPres_S1 : nesl_utility/PS-Simulink Converter  PhysicalDomain=network_engine_domain  SubClassName=ps_output  LeftPortType=input  RightPortType=output  PseudoPeriodic=off  Frequencies=[]  VectorFormat=inherit  Unit=inherit  AffineConversion=off
  aTemp_S1 : nesl_utility/PS-Simulink Converter  PhysicalDomain=network_engine_domain  SubClassName=ps_output  LeftPortType=input  RightPortType=output  PseudoPeriodic=off  Frequencies=[]  VectorFormat=inherit  Unit=degC  AffineConversion=off
  Conn1 : PMIOPort  Side=Left
  Conn2 : PMIOPort  Port=2  Side=Right
  tag scope: S8=global
  wires:
  aTemp_S1/1 -> Bus Creator/2  "aTemp_S8"
  aPres_S1/1 -> Bus Creator/1  "aPres_S8"
  Bus Creator/1 -> [S8]
  connections:
  Pressure & Temperature Sensor (G)4/LConn1 -- Conn1/RConn1 -- Conn2/RConn1
  Absolute Reference (G)/LConn1 -- Pressure & Temperature Sensor (G)4/RConn1
  aPres_S1/LConn1 -- Pressure & Temperature Sensor (G)4/RConn2
  aTemp_S1/LConn1 -- Pressure & Temperature Sensor (G)4/RConn3
